simulink model "simple_no_faults_20250727_233520"  (R2024b)
settings: Solver=ode45  StartTime=0.0  StopTime=0.01638  MaxStep=1.25e-08  RelTol=1e-3
undefined symbols (not defined in the file): sim_max_step, sim_ts
libraries: spsSeriesRLCBranchLib x7, spsDistributedParametersLineFrequencyDependentLib x6, spsGroundLib x4, spsVoltageMeasurementLib x2, spsControlledVoltageSourceLib x1, sps_lib x1
settings Model: Creator=nathanielfargo  LastModifiedBy=nathanielfargo

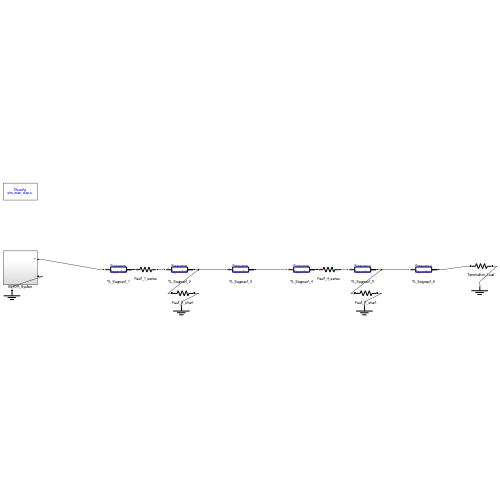
[thumbnail: Simulink's stored preview of the top-level diagram]
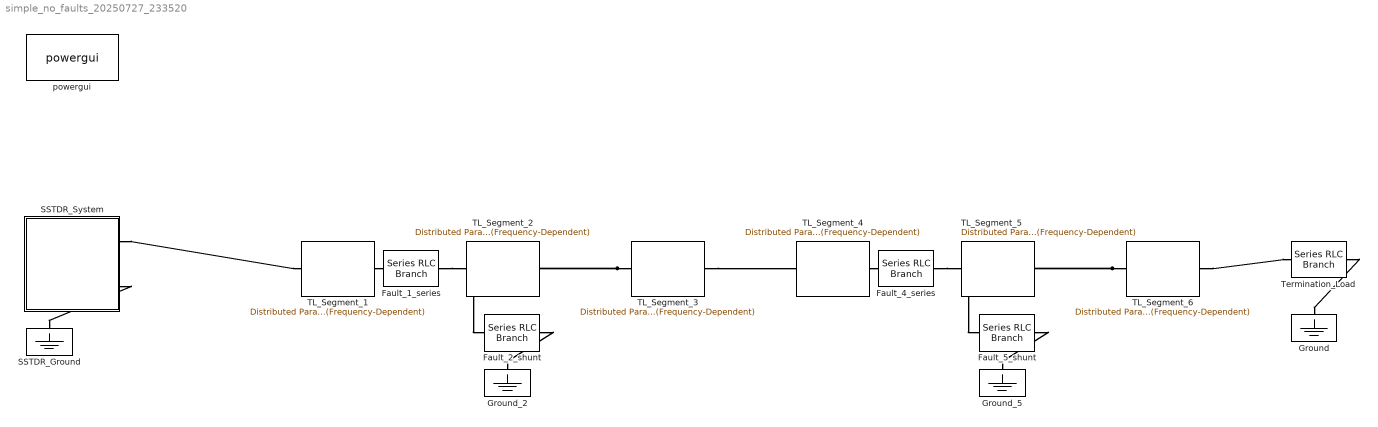
== system simple_no_faults_20250727_233520 ==
  Fault_1_series : spsSeriesRLCBranchLib/Series RLC Branch  LConnTagsString=__new0  RConnTagsString=__new0  BranchType=R  Resistance=1.1e+01  Inductance=0  SetiL0=off  InitialCurrent=0  Capacitance=inf  Setx0=off  InitialVoltage=0  Measurements=None
  Fault_2_shunt : spsSeriesRLCBranchLib/Series RLC Branch  LConnTagsString=__new0  RConnTagsString=__new0  BranchType=R  Resistance=1.9e+03  Inductance=0  SetiL0=off  InitialCurrent=0  Capacitance=inf  Setx0=off  InitialVoltage=0  Measurements=None
  Fault_4_series : spsSeriesRLCBranchLib/Series RLC Branch  LConnTagsString=__new0  RConnTagsString=__new0  BranchType=R  Resistance=2.5e+01  Inductance=0  SetiL0=off  InitialCurrent=0  Capacitance=inf  Setx0=off  InitialVoltage=0  Measurements=None
  Fault_5_shunt : spsSeriesRLCBranchLib/Series RLC Branch  LConnTagsString=__new0  RConnTagsString=__new0  BranchType=R  Resistance=2.3e+02  Inductance=0  SetiL0=off  InitialCurrent=0  Capacitance=inf  Setx0=off  InitialVoltage=0  Measurements=None
  Ground : spsGroundLib/Ground  LConnTagsString=a
  Ground_2 : spsGroundLib/Ground  LConnTagsString=a
  Ground_5 : spsGroundLib/Ground  LConnTagsString=a
  SSTDR_Ground : spsGroundLib/Ground  LConnTagsString=a
  SSTDR_System : Subsystem
  TL_Segment_{1..6} (6 alike) : spsDistributedParametersLineFrequencyDependentLib/Distributed Parameters Line (Frequency-Dependent)  WBfile=config/line_params/line_test.mat  L=1  NbPhases=1  Frange=1.00e+00 Hz to 1.00e+09 Hz, 141 points.  Comments=|  Measurements=None
      | Example of a 735 KV three-phase line
      |
      | Three bundles of 4 Bersfort ACSR 1355 MCM conductors
      | Two 1/2 inch diameter steel grounds wires
      |
      | Ytower =Ymin =  average heights of conductors
  Termination_Load : spsSeriesRLCBranchLib/Series RLC Branch  LConnTagsString=__new0  RConnTagsString=__new0  BranchType=R  Resistance=1.0e+07  Inductance=0  SetiL0=off  InitialCurrent=0  Capacitance=inf  Setx0=off  InitialVoltage=0  Measurements=None
  powergui : sps_lib/powergui  Priority=1  SimulationMode=Discrete  SampleTime=sim_max_step  frequency=60  Iterations=50  frequencyindice=0  Pbase=100e6  ErrMax=1e-4  UnitsV=kV  UnitsW=MW  buscounter=0  FunctionMessages=off  echomessages=off  EnableUseOfTLC=off  CurrentSourceSwitches=off  DisableSnubberDevices=off  DisableRonSwitches=off  DisableVfSwitches=off  DisplayEquations=off  AutomaticDiscreteSolvers=off  SolverType=Tustin/Backward Euler (TBE)  Interpol=off  ExternalGateDelay=off  methode=off  Ts=100  x0status=blocks  SPID=on  SwTol=0  HookPort=off  NonlinearTolerance=1e-4  nMaxIteration=100  ContinueOnMaxIteration=off  RestoreLinks=warning  ResistiveCurrentMeasurement=off  Frange=[0:2:500]  Ylog=off  Xlog=on  ShowGrid=off  save=off  variable=ZData  structure=0  ZoomFFT=off  StartTime=0.0  cycles=1  DisplayStyle=1  fundamental=60  FreqAxis=off  MaxFrequency=1000  frequencyindicesteady=1  RmsSteady=1  display=off
  connections:
  SSTDR_System/RConn1 -- TL_Segment_1/LConn1
  SSTDR_System/RConn2 -- SSTDR_Ground/LConn1
  TL_Segment_1/RConn1 -- Fault_1_series/LConn1
  Fault_1_series/RConn1 -- TL_Segment_2/LConn1
  TL_Segment_3/LConn1 -- TL_Segment_2/RConn1 -- Fault_2_shunt/LConn1
  TL_Segment_3/RConn1 -- TL_Segment_4/LConn1
  TL_Segment_4/RConn1 -- Fault_4_series/LConn1
  Fault_4_series/RConn1 -- TL_Segment_5/LConn1
  TL_Segment_6/LConn1 -- TL_Segment_5/RConn1 -- Fault_5_shunt/LConn1
  Fault_2_shunt/RConn1 -- Ground_2/LConn1
  Fault_5_shunt/RConn1 -- Ground_5/LConn1
  TL_Segment_6/RConn1 -- Termination_Load/LConn1
  Termination_Load/RConn1 -- Ground/LConn1

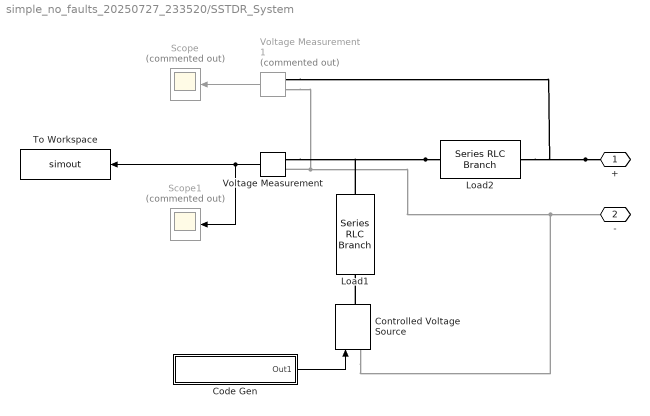
== system simple_no_faults_20250727_233520/SSTDR_System ==
  Code Gen : Subsystem
  Controlled Voltage Source : spsControlledVoltageSourceLib/Controlled Voltage Source  Initialize=on  Source_Type=DC  Amplitude=0  Phase=0  Frequency=0  Measurements=None
  Load1 : spsSeriesRLCBranchLib/Series RLC Branch  LConnTagsString=__new0  RConnTagsString=__new0  BranchType=L  Resistance=25  Inductance=100e-6  SetiL0=off  InitialCurrent=0  Capacitance=1e-6  Setx0=off  InitialVoltage=0  Measurements=None
  Load2 : spsSeriesRLCBranchLib/Series RLC Branch  LConnTagsString=__new0  RConnTagsString=__new0  BranchType=C  Resistance=0  Inductance=0  SetiL0=off  InitialCurrent=0  Capacitance=1e-6  Setx0=off  InitialVoltage=0  Measurements=None
  Scope : Scope  Commented=on
  Scope1 : Scope  Commented=on
  To Workspace : ToWorkspace  VariableName=simout  SaveFormat=Structure With Time  SampleTime=sim_ts
  Voltage Measurement : spsVoltageMeasurementLib/Voltage Measurement  PhasorSimulation=off  OutputType=Complex  PSBequivalent=0
  Voltage Measurement1 : spsVoltageMeasurementLib/Voltage Measurement  Commented=on  PhasorSimulation=off  OutputType=Complex  PSBequivalent=0
  + : PMIOPort  Side=Right
  - : PMIOPort  Port=2  Side=Right
  wires:
  Voltage Measurement1/1 -> Scope/1
  Voltage Measurement/1 -> To Workspace/1, Scope1/1
  Code Gen/1(Out1) -> Controlled Voltage Source/1
  connections:
  +/RConn1 -- Voltage Measurement1/LConn1 -- Load2/RConn1
  Voltage Measurement1/LConn2 -- -/RConn1 -- Controlled Voltage Source/LConn1 -- Voltage Measurement/LConn2
  Load2/LConn1 -- Load1/RConn1 -- Voltage Measurement/LConn1
  Controlled Voltage Source/RConn1 -- Load1/LConn1

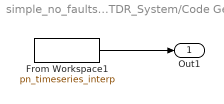
== system simple_no_faults_20250727_233520/SSTDR_System/Code Gen ==
  From Workspace1 : FromWorkspace  VariableName=pn_timeseries_interp  OutputAfterFinalValue=Setting to zero
  Out1 : Outport
  wires:
  From Workspace1/1 -> Out1/1
